simulink subsystem "no_wave"  (R2025b)
settings: Solver=VariableStepAuto  StartTime=0.0  StopTime=10.0  RelTol=1e-3
settings Model: Creator=sanborkl

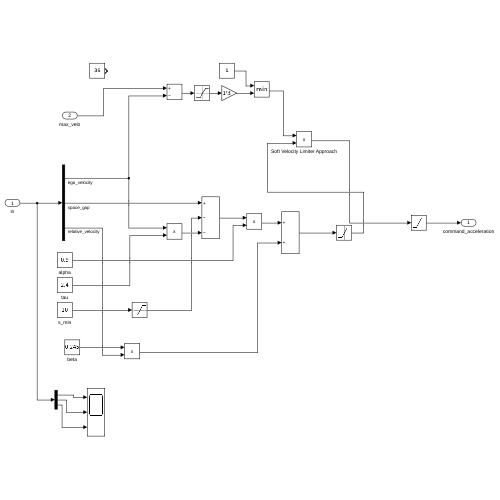
[thumbnail: Simulink's stored preview of the top-level diagram]
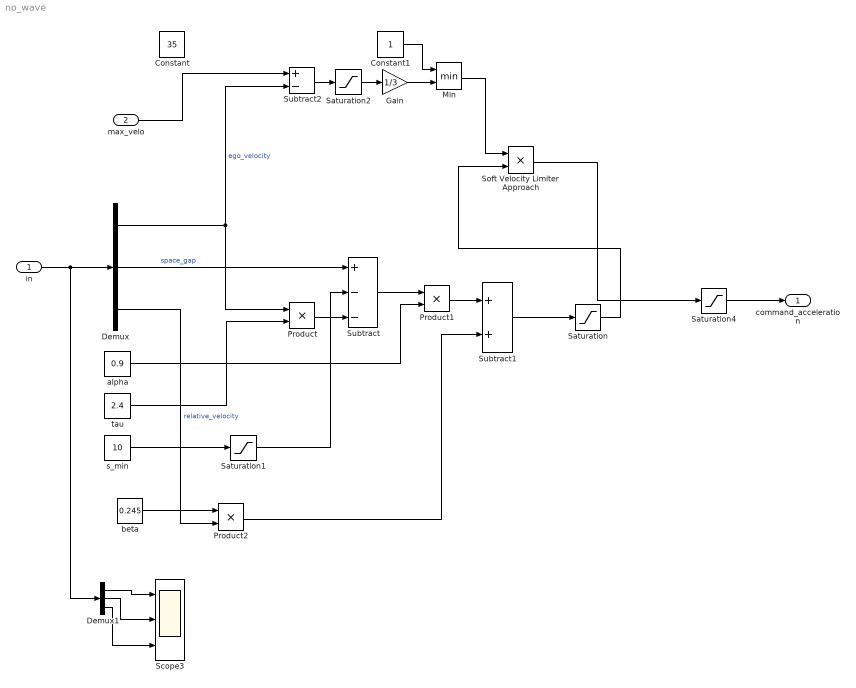
== system no_wave ==
  in : Inport
  max_velo : Inport  Port=2
  Constant : Constant  Value=35
  Constant1 : Constant
  Demux : Demux  Outputs=3
  Demux1 : Demux  Outputs=3
  Gain : Gain  Gain=1/3
  Min : MinMax  Inputs=2
  Product : Product
  Product1 : Product
  Product2 : Product
  Saturation : Saturate  UpperLimit=1.5  LowerLimit=-3
  Saturation1 : Saturate  UpperLimit=500  LowerLimit=5
  Saturation2 : Saturate  UpperLimit=3  LowerLimit=0
  Saturation4 : Saturate  UpperLimit=1.5  LowerLimit=-3
  Scope3 : Scope  NumInputPorts=3
      settings: ActiveDisplayYMinimum=-1  ActiveDisplayYMaximum=1  DataLoggingVariableName=ScopeData13
  Soft Velocity Limiter Approach : Product
  Subtract : Sum  Inputs=+--
  Subtract1 : Sum
  Subtract2 : Sum  Inputs=+-
  alpha : Constant  Value=0.9
  beta : Constant  Value=0.245
  s_min : Constant  Value=10
  tau : Constant  Value=2.4
  command_acceleration : Outport
  wires:
  Demux/3 -> Product2/2  "relative_velocity"
  Product/1 -> Subtract/3
  Subtract/1 -> Product1/1
  tau/1 -> Product/2
  Demux/1 -> Product/1, Subtract2/2  "ego_velocity"
  Demux/2 -> Subtract/1  "space_gap"
  s_min/1 -> Saturation1/1
  alpha/1 -> Product1/2
  Saturation1/1 -> Subtract/2
  Demux1/3 -> Scope3/3
  Demux1/2 -> Scope3/2
  Demux1/1 -> Scope3/1
  in/1 -> Demux/1, Demux1/1
  beta/1 -> Product2/1
  Product1/1 -> Subtract1/1
  Subtract2/1 -> Saturation2/1
  Saturation2/1 -> Gain/1
  Gain/1 -> Min/2
  Constant1/1 -> Min/1
  Min/1 -> Soft Velocity Limiter Approach/1
  Subtract1/1 -> Saturation/1
  Saturation4/1 -> command_acceleration/1
  Saturation/1 -> Soft Velocity Limiter Approach/2
  Product2/1 -> Subtract1/2
  Soft Velocity Limiter Approach/1 -> Saturation4/1
  max_velo/1 -> Subtract2/1
